simulink model "Fig430"  (R2014b)
settings: Solver=ode3  StartTime=0.0  StopTime=.005  FixedStep=1.5625e-6  RelTol=1e-3
libraries: dspsigops x13, dspquant2 x2, commutil2 x1, dsparch4 x1
settings Model: DataTypeOverride=Double  MinMaxOverflowLogging=ForceOff  Creator=Dennis Silage  LastModifiedBy=Silage
settings DataIOCC: SignalLoggingSaveFormat=ModelDataLogs
settings OptimizationCC: ExpressionDepthLimit=2147483647  InitFltsAndDblsToZero=on
settings DebuggingCC: UnderspecifiedInitializationDetection=Classic  MergeDetectMultiDrivingBlocksExec=none  FcnCallInpInsideContextMsg=UseLocalSettings  UnconnectedOutputMsg=none  StateNameClashWarn=warning
settings GRTTargetCC: CombineOutputUpdateFcns=off  GRTInterface=on

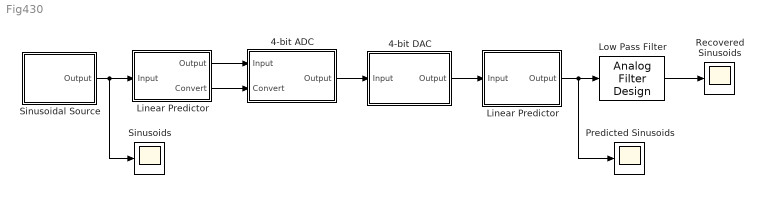
== system Fig430 ==
  4-bit ADC : Subsystem
  4-bit DAC : Subsystem
  Linear Predictor : Subsystem
  "Linear Predictor " : Subsystem
  Low Pass Filter : dsparch4/Analog Filter Design  method=Butterworth  filttype=Lowpass  N=9  Wlo=7500*pi  Whi=80  Rp=2  Rs=40
  Predicted Sinusoids : Scope
      settings: YMin=-1.5  YMax=1.5
  Recovered Sinusoids : Scope
      settings: YMin=-1.5  YMax=1.5  SaveName=ScopeData4
  Sinusoidal Source : Subsystem
  Sinusoids : Scope
      settings: YMin=-1.5  YMax=1.5  SaveName=ScopeData2
  wires:
  4-bit DAC/1(Output) -> "Linear Predictor "/1(Input)
  Low Pass Filter/1 -> Recovered Sinusoids/1
  "Linear Predictor "/1(Output) -> Predicted Sinusoids/1, Low Pass Filter/1
  Sinusoidal Source/1(Output) -> Linear Predictor/1(Input), Sinusoids/1
  Linear Predictor/1(Output) -> 4-bit ADC/1(Input)
  Linear Predictor/2(Convert) -> 4-bit ADC/2("Convert  ")
  4-bit ADC/1(Output) -> 4-bit DAC/1(Input)

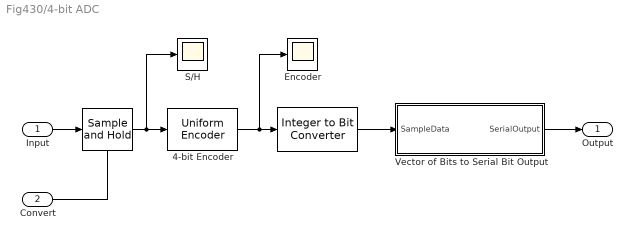
== system Fig430/4-bit ADC ==
  Input : Inport
  "Convert  " : Inport  Port=2
  " " : commutil2/Integer to Bit Converter  nbits=4  signedInputValues=Unsigned  bitOrder=LSB first  outDtype=uint8
  "   " : dspsigops/Sample and Hold  trig=Rising edge  initCond=0  latchinput=off
  4-bit Encoder : dspquant2/Uniform Encoder  peak=2.56  bits=4  otype=Unsigned integer
  Encoder : Scope
      settings: YMin=-10  YMax=20  SaveName=ScopeData3
  S/H : Scope
      settings: YMin=-2.5  YMax=2.5  SaveName=ScopeData6
  Vector of Bits to Serial Bit Output : MATLAB Function  TreatAsAtomicUnit=on
  Output : Outport
  wires:
  " "/1 -> Vector of Bits to Serial Bit Output/1(SampleData)
  4-bit Encoder/1 -> " "/1, Encoder/1
  Vector of Bits to Serial Bit Output/1(SerialOutput) -> Output/1
  Input/1 -> "   "/1
  "Convert  "/1 -> "   "/Trigger
  "   "/1 -> S/H/1, 4-bit Encoder/1

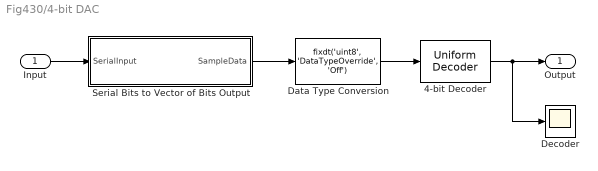
== system Fig430/4-bit DAC ==
  Input : Inport
  4-bit Decoder : dspquant2/Uniform Decoder  peak=2.56  bits=4  overflowMode=Saturate  otype=Double
  Data Type Conversion : DataTypeConversion  OutDataTypeStr=fixdt('uint8', 'DataTypeOverride', 'Off')  LockScale=on
  Decoder : Scope
      settings: YMin=-1.5  YMax=1.5  SaveName=ScopeData5
  Serial Bits to Vector of Bits Output : MATLAB Function  TreatAsAtomicUnit=on
  Output : Outport
  wires:
  Data Type Conversion/1 -> 4-bit Decoder/1
  Serial Bits to Vector of Bits Output/1(SampleData) -> Data Type Conversion/1
  4-bit Decoder/1 -> Output/1, Decoder/1
  Input/1 -> Serial Bits to Vector of Bits Output/1(SerialInput)

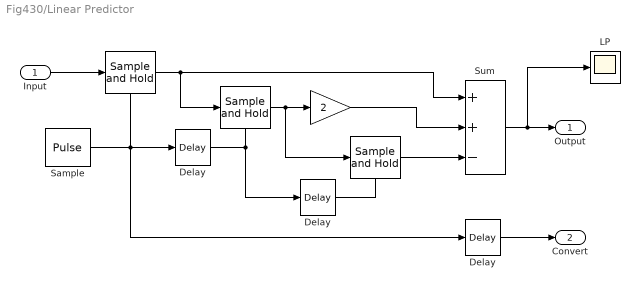
== system Fig430/Linear Predictor ==
  Input : Inport
  "   " : dspsigops/Sample and Hold  trig=Rising edge  initCond=0  latchinput=off
  "    " : dspsigops/Sample and Hold  trig=Rising edge  initCond=0  latchinput=off
  "      " : dspsigops/Sample and Hold  trig=Rising edge  initCond=0  latchinput=off
  "           " : Gain  Gain=2
  " Delay  " : dspsigops/Delay  InputProcessing=Inherited (this choice will be removed - see release notes)  dly_unit=Samples  delay=80  ic_detail=off  dif_ic_for_ch=off  dif_ic_for_dly=off  ic=0  reset_popup=None
  Delay : dspsigops/Delay  InputProcessing=Inherited (this choice will be removed - see release notes)  dly_unit=Samples  delay=40  ic_detail=off  dif_ic_for_ch=off  dif_ic_for_dly=off  ic=0  reset_popup=None
  "Delay " : dspsigops/Delay  InputProcessing=Inherited (this choice will be removed - see release notes)  dly_unit=Samples  delay=78  ic_detail=off  dif_ic_for_ch=off  dif_ic_for_dly=off  ic=0  reset_popup=None
  LP : Scope
      settings: YMin=-2.5  YMax=2.5
  Sample : DiscretePulseGenerator  PulseType=Time based  Period=1.25e-4  PulseWidth=10  SampleTime=1.25e-6
  Sum : Sum  Inputs=++-
  Output : Outport
  Convert : Outport  Port=2
  wires:
  Input/1 -> "   "/1
  Sum/1 -> LP/1, Output/1
  "   "/1 -> Sum/1, "    "/1
  "    "/1 -> "      "/1, "           "/1
  "           "/1 -> Sum/2
  "      "/1 -> Sum/3
  "Delay "/1 -> " Delay  "/1, "    "/Trigger
  " Delay  "/1 -> "      "/Trigger
  Sample/1 -> Delay/1, "   "/Trigger, "Delay "/1
  Delay/1 -> Convert/1

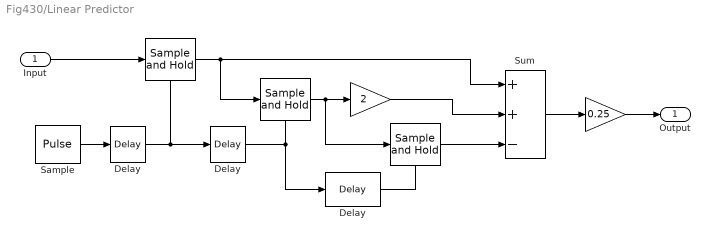
== system Fig430/Linear Predictor  ==
  Input : Inport
  "  " : dspsigops/Sample and Hold  trig=Rising edge  initCond=0  latchinput=off
  "   " : dspsigops/Sample and Hold  trig=Rising edge  initCond=0  latchinput=off
  "    " : dspsigops/Sample and Hold  trig=Rising edge  initCond=0  latchinput=off
  "          " : Gain  Gain=0.25
  "           " : Gain  Gain=2
  "   Delay  " : dspsigops/Delay  InputProcessing=Inherited (this choice will be removed - see release notes)  dly_unit=Samples  delay=120  ic_detail=off  dif_ic_for_ch=off  dif_ic_for_dly=off  ic=0  reset_popup=None
  "  Delay " : dspsigops/Delay  InputProcessing=Inherited (this choice will be removed - see release notes)  dly_unit=Samples  delay=38  ic_detail=off  dif_ic_for_ch=off  dif_ic_for_dly=off  ic=0  reset_popup=None
  Delay : dspsigops/Delay  InputProcessing=Inherited (this choice will be removed - see release notes)  dly_unit=Samples  delay=40  ic_detail=off  dif_ic_for_ch=off  dif_ic_for_dly=off  ic=0  reset_popup=None
  Sample : DiscretePulseGenerator  PulseType=Time based  Period=1.25e-4  PulseWidth=10  SampleTime=1.25e-6
  Sum : Sum  Inputs=++-
  Output : Outport
  wires:
  Input/1 -> "   "/1
  "   "/1 -> Sum/1, "    "/1
  "    "/1 -> "  "/1, "           "/1
  "           "/1 -> Sum/2
  "  "/1 -> Sum/3
  "  Delay "/1 -> "    "/Trigger, "   Delay  "/1
  "   Delay  "/1 -> "  "/Trigger
  Sample/1 -> Delay/1
  Delay/1 -> "   "/Trigger, "  Delay "/1
  Sum/1 -> "          "/1
  "          "/1 -> Output/1

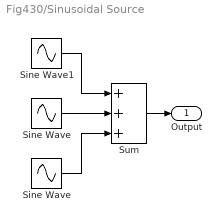
== system Fig430/Sinusoidal Source ==
  " Sine Wave " : Sin  Amplitude=0.2  Frequency=5000*pi  SampleTime=1.5625e-6
  "Sine Wave " : Sin  Amplitude=0.5  Frequency=3000*pi  SampleTime=1.5625e-6
  Sine Wave1 : Sin  Frequency=1000*pi  SampleTime=1.5625e-6
  Sum : Sum  Inputs=+++
  Output : Outport
  wires:
  "Sine Wave "/1 -> Sum/2
  " Sine Wave "/1 -> Sum/3
  Sine Wave1/1 -> Sum/1
  Sum/1 -> Output/1

== matlab function Fig430/4-bit DAC/Serial Bits to Vector of Bits Output ==
  data: SerialInput input; SampleData output
function SampleData = fcn(SerialInput)
%#codegen

persistent SmpDat  SmpNum SmpDatOld

if isempty(SmpNum)
    SmpNum = 0;
    SmpDat = 0;
    SmpDatOld = 0;
    SampleData = 0;
end

SmpNum = SmpNum + 1;
if (SmpNum == 5)
    SmpNum = 1;
    SampleData = SmpDat;
    SmpDatOld = SmpDat;
    SmpDat = SerialInput;
else
    SampleData = SmpDatOld;
    SmpDat = SmpDat + SerialInput*2^(SmpNum-1);
end

end

== matlab function Fig430/4-bit ADC/Vector of Bits to Serial Bit Output ==
  data: SampleData input; SerialOutput output
function SerialOutput = fcn(SampleData)
%#codegen
persistent SmpDat SmpNum

if isempty(SmpNum)
    SmpNum = 1;
    SmpDat = SampleData;
end

SerialOutput = SampleData(SmpNum);
SmpNum = SmpNum + 1;
if (SmpNum == 5)
    SmpNum = 1;
    SmpDat = SampleData;
end

end
